simulink model "b747_front_land_gear_sim"  (R2023b)
settings: Solver=VariableStepAuto  StartTime=0.0  StopTime=30  RelTol=1e-6
values from neighbouring files (symbols this model uses):
  Q = force(X, Y)    [sas_loads.m]
  velocity = linspace(50, 150, 100)    [sas_loads.m]
  x = linspace(0, 0.146, 1000)    [b747_front_land_gear.m]    (also in sas_aero.m = linspace(0, 1.57, 100); sas_dumper.m = alpha * 360 / 2 / pi; sas_weight.m = linspace(0, 1.57, 100))
  y = gear_angle(x)    [b747_front_land_gear.m]    (also in sas_aero.m = 1:100; sas_dumper.m = M; sas_weight.m = 1:100)
libraries: simulink x2, slpidlib x1, SignalEditorBlockLib x1
settings Model: Creator=bohdan  LastModifiedBy=bohdan

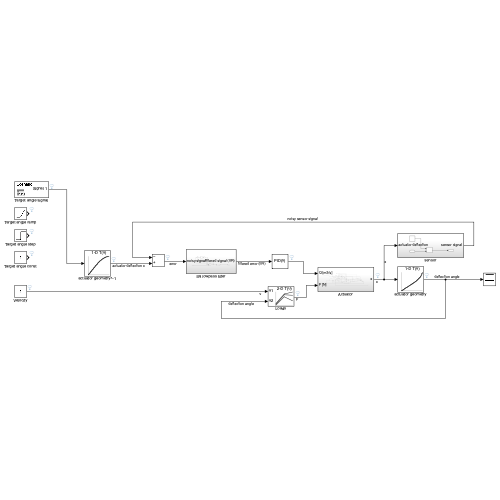
[thumbnail: Simulink's stored preview of the top-level diagram]
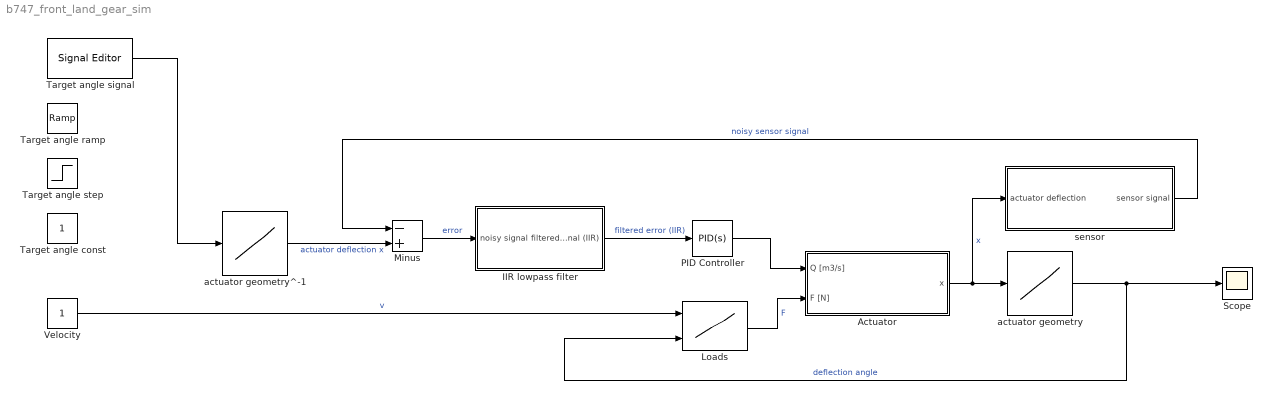
== system b747_front_land_gear_sim ==
  Actuator : Subsystem
  IIR lowpass filter : Subsystem
  Loads : Lookup_n-D  BreakpointsForDimension1=velocity  BreakpointsForDimension2=angle  Table=Q  InternalRulePriority=Speed  RndMeth=Simplest
      settings: InputPortMap=u0,u1
  Minus : Sum  Inputs=-+
  PID Controller : slpidlib/PID Controller  Controller=PID  Form=Parallel  TimeDomain=Continuous-time  UseExternalTs=off  SampleTime=-1  IntegratorMethod=Forward Euler  FilterMethod=Forward Euler  ControllerParametersSource=internal  P=0.011  I=0  UseKiTs=off  D=0.0015  N=100  UseFilter=on  TunerSelectOption=Transfer Function Based (PID Tuner App)  InitialConditionSource=internal  InitialConditionForIntegrator=0  InitialConditionForFilter=0  DifferentiatorICPrevScaledInput=0  ExternalReset=none  TrackingMode=off  Kt=1  LimitOutput=off  SatLimitsSource=internal  UpperSaturationLimit=inf  LowerSaturationLimit=-inf  LinearizeAsGain=on  AntiWindupMode=none  Kb=1  LimitIntegrator=off  UpperIntegratorSaturationLimit=inf  LowerIntegratorSaturationLimit=-inf  POutMin=[]  POutMax=[]  IOutMin=[]  IOutMax=[]  DOutMin=[]  DOutMax=[]  NOutMin=[]  NOutMax=[]  SumOutMin=[]  SumOutMax=[]  SaturationOutMin=[]  SaturationOutMax=[]  PParamMin=[]  PParamMax=[]  IParamMin=[]  IParamMax=[]  DParamMin=[]  DParamMax=[]  NParamMin=[]  NParamMax=[]  KbParamMin=[]  KbParamMax=[]  KtParamMin=[]  KtParamMax=[]  KbOutMin=[]  KbOutMax=[]  KtOutMin=[]  KtOutMax=[]  IntegratorOutMin=[]  IntegratorOutMax=[]  FilterOutMin=[]  FilterOutMax=[]  SumI1OutMin=[]  SumI1OutMax=[]  SumI2OutMin=[]  SumI2OutMax=[]  SumI3OutMin=[]  SumI3OutMax=[]  SumI4OutMin=[]  SumI4OutMax=[]  SumDOutMin=[]  SumDOutMax=[]  DifferentiatorOutMin=[]  DifferentiatorOutMax=[]  FilterDiffOutCoefMin=[]  FilterDiffOutCoefMax=[]  ReciprocalOutMin=[]  ReciprocalOutMax=[]  SumDenOutMin=[]  SumDenOutMax=[]  SumNumOutMin=[]  SumNumOutMax=[]  DivideOutMin=[]  DivideOutMax=[]  UdiffTsProdOutMin=[]  UdiffTsProdOutMax=[]  NTsProdOutMin=[]  NTsProdOutMax=[]  UintegralTsProdOutMin=[]  UintegralTsProdOutMax=[]  UngainTsProdOutMin=[]  UngainTsProdOutMax=[]  ClampingZeroOutDataTypeStr=Inherit: Inherit via back propagation  ClampingZeroOutMin=[]  ClampingZeroOutMax=[]  FilterDenConstantOutDataTypeStr=Inherit: Inherit via back propagation  FilterDenConstantOutMin=[]  FilterDenConstantOutMax=[]  PCopyOutDataTypeStr=Inherit: Inherit via back propagation  PCopyOutMin=[]  PCopyOutMax=[]  NCopyOutDataTypeStr=Inherit: Inherit via back propagation  NCopyOutMin=[]  NCopyOutMax=[]  IntegratorContinuousStateAttributes=''  IntegratorStateMustResolveToSignalObject=off  IntegratorRTWStateStorageClass=Auto  FilterContinuousStateAttributes=''  FilterStateMustResolveToSignalObject=off  FilterRTWStateStorageClass=Auto  ParallelPVariant=InternalParameters  IdealPVariant=Disabled  IVariant=InternalParameters  DVariant=InternalParameters  IntegratorVariant=Continuous  SatVariant=Disabled  AWVariant=Passthrough  PCopyVariant=Disabled  TRVariant=Disabled  FdbkBlocksVariant=Forward  IdealPFdbkVariant=Disabled  SatFdbkVariant=Disabled  DerivativeFilterVariant=ContFilter  NVariant=InternalParameters  NCopyVariant=Disabled  FilterICVariant=InternalICsFilter  IntegratorICVariant=InternalICs  ExternalResetVariant=Disabled  TRSumVariant=Passthrough  SumFdbkVariant=Disabled  SumVariant=Sum_PID  TsampFilterVariant=InternalTs  TsampNgainVariant=Passthrough  TsampIntegralVariant=Disabled_SignalSpec  ExternalSaturationOutDataTypeStr=Inherit: Same as second input
  Scope : Scope
  Target angle const : Constant
  Target angle ramp : simulink/Sources/Ramp  slope=1  start=0  InitialOutput=0
  Target angle signal : SignalEditorBlockLib/Signal Editor  FileName=steps.mat  ActiveScenario=Scenario  ActiveSignal=Signal 1  IsBus=off  OutputBusObjectStr=Bus: BusObject  SampleTime=0  Interpolate=off  ZeroCross=off  OutputAfterFinalValue=Setting to zero  Unit=inherit  PreserveSignalName=on  ApplySigPropsToAllScenarios=on  ApplySigPropsToAllSignals=off
  Target angle step : Step  After=1.57  SampleTime=0
  Velocity : Constant
  actuator geometry : Lookup_n-D  NumberOfTableDimensions=1  BreakpointsForDimension1=x  Table=y  InternalRulePriority=Speed  RndMeth=Simplest
  actuator geometry^-1 : Lookup_n-D  NumberOfTableDimensions=1  BreakpointsForDimension1=y  Table=x  InternalRulePriority=Speed  RndMeth=Simplest
  sensor : Subsystem
  wires:
  Velocity/1 -> Loads/1  "v"
  actuator geometry/1 -> Loads/2, Scope/1  "deflection angle"
  Loads/1 -> Actuator/2(F [N])  "F"
  Actuator/1(x) -> sensor/1(actuator deflection), actuator geometry/1  "x"
  PID Controller/1 -> Actuator/1(Q [m3/s])
  actuator geometry^-1/1 -> Minus/2  "actuator deflection x"
  Minus/1 -> IIR lowpass filter/1(noisy signal)  "error"
  IIR lowpass filter/1(filtered signal (IIR)) -> PID Controller/1  "filtered error (IIR)"
  sensor/1(sensor signal) -> Minus/1  "noisy sensor signal"
  Target angle signal/1 -> actuator geometry^-1/1

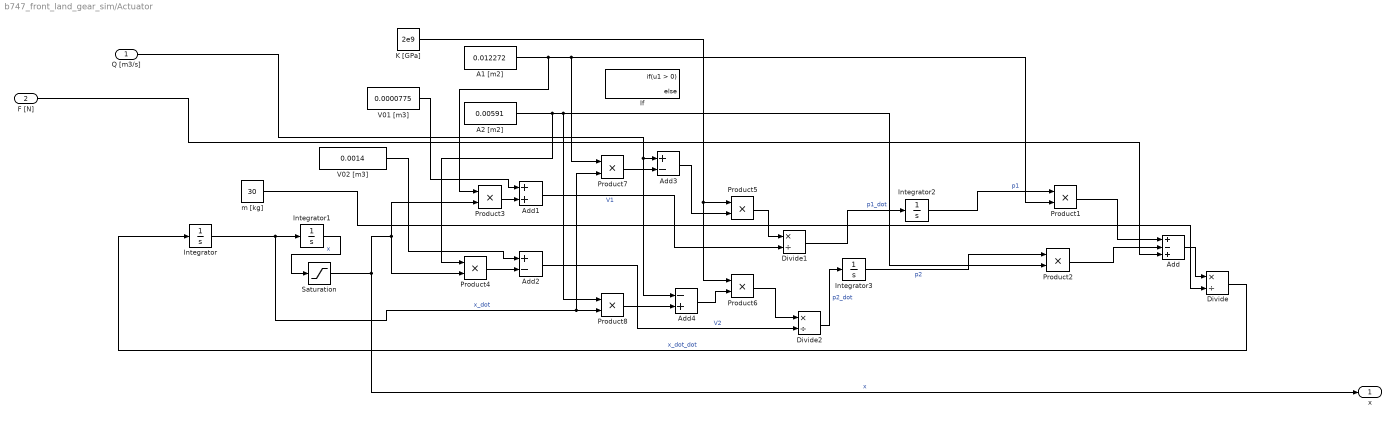
== system b747_front_land_gear_sim/Actuator ==
  Q [m3/s] : Inport
  F [N] : Inport  Port=2
  A1 [m2] : Constant  Value=0.012272
  A2 [m2] : Constant  Value=0.00591
  Add : Sum  Inputs=+-+
  Add1 : Sum
  Add2 : Sum  Inputs=+-
  Add3 : Sum  Inputs=+-
  Add4 : Sum  Inputs=-+
  Divide : Product  Inputs=*/
  Divide1 : Product  Inputs=*/
  Divide2 : Product  Inputs=*/
  If : If
  Integrator : Integrator
  Integrator1 : Integrator
  Integrator2 : Integrator  InitialCondition=1e5
  Integrator3 : Integrator  InitialCondition=1e5
  K [GPa] : Constant  Value=2e9
  Product{1..8} (8 alike) : Product
  Saturation : Saturate  UpperLimit=0.2  LowerLimit=0
  V01 [m3] : Constant  Value=0.0000775
  V02 [m3] : Constant  Value=0.0014
  m [kg] : Constant  Value=30
  x : Outport
  wires:
  m [kg]/1 -> Divide/2
  Add2/1 -> Divide2/2  "V2"
  K [GPa]/1 -> Product6/1, Product5/1
  F [N]/1 -> Add/3
  Product6/1 -> Divide2/1
  Product7/1 -> Add3/2
  Product2/1 -> Add/2
  Add1/1 -> Divide1/2  "V1"
  V02 [m3]/1 -> Add2/1
  Product5/1 -> Divide1/1
  Divide/1 -> Integrator/1  "x_dot_dot"
  A2 [m2]/1 -> Product4/1, Product8/1, Product2/2
  Product1/1 -> Add/1
  Divide2/1 -> Integrator3/1  "p2_dot"
  Product3/1 -> Add1/2
  Divide1/1 -> Integrator2/1  "p1_dot"
  A1 [m2]/1 -> Product3/1, Product7/1, Product1/2
  Add3/1 -> Product5/2
  Product8/1 -> Add4/2
  Add4/1 -> Product6/2
  V01 [m3]/1 -> Add1/1
  Integrator/1 -> Product7/2, Product8/2, Integrator1/1  "x_dot"
  Integrator2/1 -> Product1/1  "p1"
  Q [m3/s]/1 -> Add4/1, Add3/1
  Product4/1 -> Add2/2
  Add/1 -> Divide/1
  Saturation/1 -> Product4/2, Product3/2, x/1  "x"
  Integrator3/1 -> Product2/1  "p2"
  Integrator1/1 -> Saturation/1  "x"

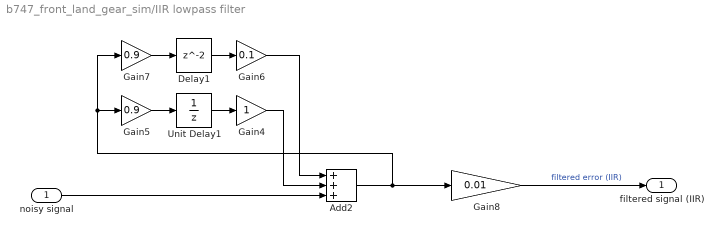
== system b747_front_land_gear_sim/IIR lowpass filter ==
  noisy signal : Inport
  Add2 : Sum  Inputs=+++
  Delay1 : Delay
  Gain4 : Gain
  Gain5 : Gain  Gain=0.9
  Gain6 : Gain  Gain=0.1
  Gain7 : Gain  Gain=0.9
  Gain8 : Gain  Gain=0.01
  Unit Delay1 : UnitDelay  SampleTime=-1  HasFrameUpgradeWarning=on
  filtered signal (IIR) : Outport
  wires:
  Gain6/1 -> Add2/1
  noisy signal/1 -> Add2/3
  Unit Delay1/1 -> Gain4/1
  Delay1/1 -> Gain6/1
  Gain4/1 -> Add2/2
  Gain8/1 -> filtered signal (IIR)/1  "filtered error (IIR)"
  Add2/1 -> Gain8/1, Gain5/1, Gain7/1
  Gain7/1 -> Delay1/1
  Gain5/1 -> Unit Delay1/1

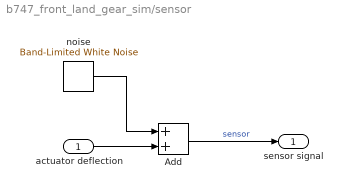
== system b747_front_land_gear_sim/sensor ==
  actuator deflection : Inport
  Add : Sum
  noise : simulink/Sources/Band-Limited White Noise  Cov=[0.00000001]  Ts=0.005  seed=[23341]
  sensor signal : Outport
  wires:
  Add/1 -> sensor signal/1  "sensor"
  actuator deflection/1 -> Add/2
  noise/1 -> Add/1
